simulink model "aperiodic1"  (R2016a)
settings: Solver=VariableStepAuto  StartTime=0.0  StopTime=10.0  RelTol=1e-3
settings Model: Creator=Jann dan Jursus  LastModifiedBy=Jann dan Jursus

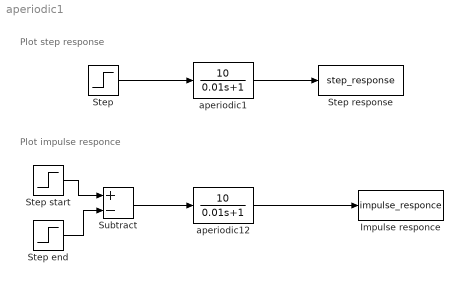
== system aperiodic1 ==
  note: Plot impulse responce
  note: Plot step response
  Impulse responce : ToWorkspace  VariableName=impulse_responce  SaveFormat=Timeseries  SampleTime=-1
  Step : Step  Time=0  SampleTime=0
  Step end : Step  Time=1.001  After=100  SampleTime=0
  Step response : ToWorkspace  VariableName=step_response  SaveFormat=Timeseries  SampleTime=-1
  Step start : Step  After=100  SampleTime=0
  Subtract : Sum  Inputs=+-
  aperiodic1 : TransferFcn  Numerator=[10]  Denominator=[0.01 1]
  aperiodic12 : TransferFcn  Numerator=[10]  Denominator=[0.01 1]
  wires:
  Step start/1 -> Subtract/1
  Step end/1 -> Subtract/2
  Subtract/1 -> aperiodic12/1
  Step/1 -> aperiodic1/1
  aperiodic1/1 -> Step response/1
  aperiodic12/1 -> Impulse responce/1
